simulink model "ModeloHibrido"  (R2023b)
settings: Solver=VariableStepAuto  StartTime=0.0  StopTime=10.0  RelTol=1e-3
settings Model: Creator=johan  LastModifiedBy=Carlos

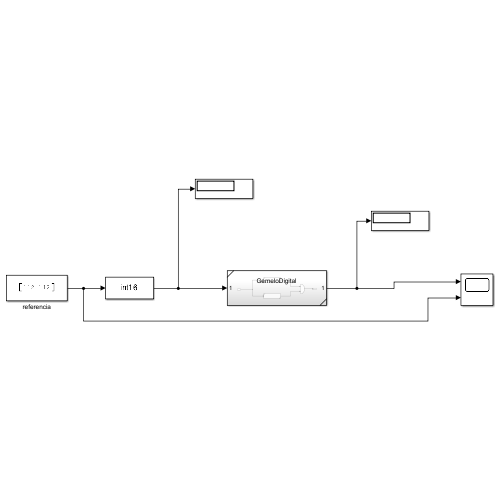
[thumbnail: Simulink's stored preview of the top-level diagram]
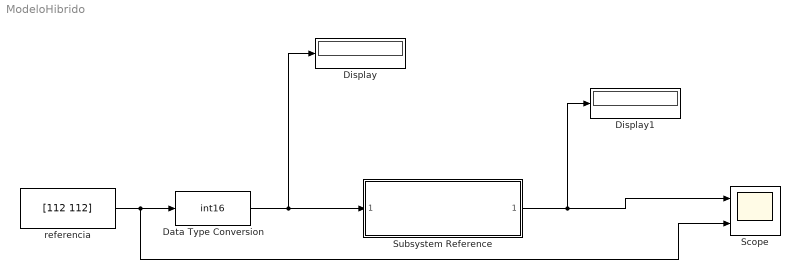
== system ModeloHibrido ==
  Data Type Conversion : DataTypeConversion  OutDataTypeStr=int16  SaturateOnIntegerOverflow=off  RndMeth=Floor
  Display : Display
  Display1 : Display
  Scope : Scope  NumInputPorts=2
  Subsystem Reference : Subsystem  ReferencedSubsystem=GemeloDigital
  referencia : Constant  Value=[112 112]
  wires:
  referencia/1 -> Scope/2, Data Type Conversion/1
  Data Type Conversion/1 -> Display/1, Subsystem Reference/1
  Subsystem Reference/1 -> Display1/1, Scope/1
